simulink model "AFO_Hopf__sim1"  (R2020a)
settings: Solver=ode4  StartTime=0.0  StopTime=20  FixedStep=0.01  RelTol=1e-3
PreLoadFcn:
  | addpath(genpath('./DMP_AFO_simulink'), genpath('./my_util'))
libraries: simulink x1
settings Model: Creator=12927  LastModifiedBy=12927

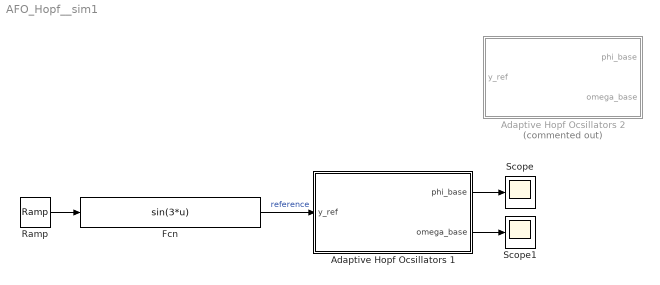
== system AFO_Hopf__sim1 ==
  Adaptive Hopf Ocsillators 1 : Subsystem
  Adaptive Hopf Ocsillators 2 : Subsystem  Commented=on
  Fcn : Fcn  Expr=sin(3*u)
  Ramp : simulink/Sources/Ramp  slope=1  start=0  InitialOutput=0
  Scope : Scope
  Scope1 : Scope
  wires:
  Ramp/1 -> Fcn/1
  Fcn/1 -> Adaptive Hopf Ocsillators 1/1(y_ref)  "reference"
  Adaptive Hopf Ocsillators 1/1(phi_base) -> Scope/1
  Adaptive Hopf Ocsillators 1/2(omega_base) -> Scope1/1

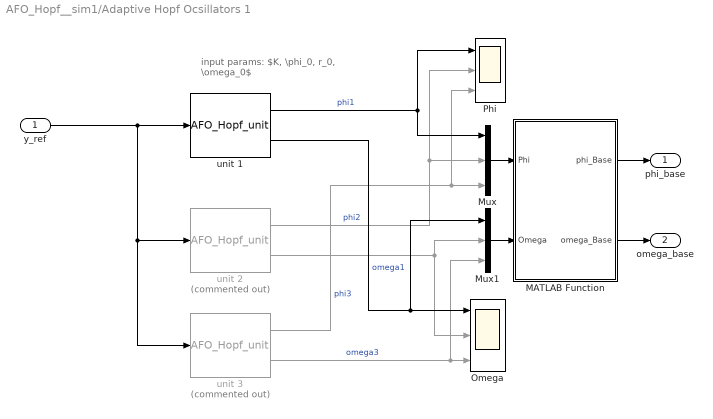
== system AFO_Hopf__sim1/Adaptive Hopf Ocsillators 1 ==
  note: input params:
      | $K, \phi_0, r_0, \omega_0$
  y_ref : Inport
  MATLAB Function : MATLAB Function  TreatAsAtomicUnit=on
  Mux : Mux  Inputs=3
  Mux1 : Mux  Inputs=3
  Omega : Scope  NumInputPorts=3
  Phi : Scope  NumInputPorts=3
  unit 1 : M-S-Function  FunctionName=AFO_Hopf_unit  Parameters=2,0,1,1
  unit 2 : M-S-Function  Commented=on  FunctionName=AFO_Hopf_unit  Parameters=10,0,1,1
  unit 3 : M-S-Function  Commented=on  FunctionName=AFO_Hopf_unit  Parameters=10,0,2,1
  phi_base : Outport
  omega_base : Outport  Port=2
  wires:
  unit 3/2 -> Omega/3, Mux1/3  "omega3"
  MATLAB Function/1(phi_Base) -> phi_base/1
  unit 2/1 -> Phi/2, Mux/2  "phi2"
  unit 2/2 -> Omega/2, Mux1/2
  Mux/1 -> MATLAB Function/1(Phi)
  unit 3/1 -> Mux/3, Phi/3  "phi3"
  Mux1/1 -> MATLAB Function/2(Omega)
  unit 1/1 -> Mux/1, Phi/1  "phi1"
  unit 1/2 -> Omega/1, Mux1/1  "omega1"
  MATLAB Function/2(omega_Base) -> omega_base/1
  y_ref/1 -> unit 1/1, unit 2/1, unit 3/1

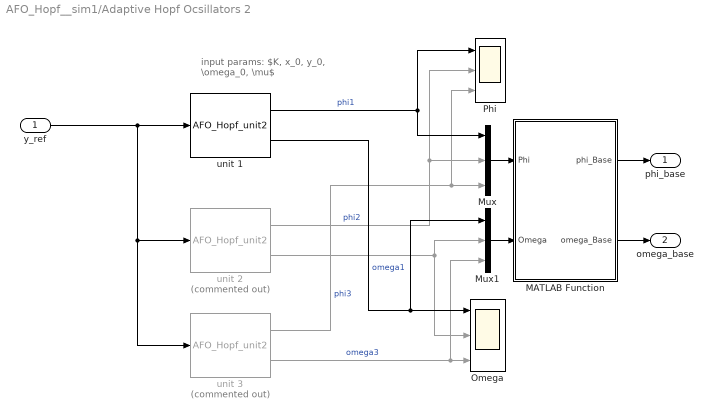
== system AFO_Hopf__sim1/Adaptive Hopf Ocsillators 2 ==
  note: input params:
      | $K, x_0, y_0, \omega_0, \mu$
  y_ref : Inport
  MATLAB Function : MATLAB Function  TreatAsAtomicUnit=on
  Mux : Mux  Inputs=3
  Mux1 : Mux  Inputs=3
  Omega : Scope  NumInputPorts=3
  Phi : Scope  NumInputPorts=3
  unit 1 : M-S-Function  FunctionName=AFO_Hopf_unit2  Parameters=5,1,0,1,1
  unit 2 : M-S-Function  Commented=on  FunctionName=AFO_Hopf_unit2  Parameters=5,1,0,1,1
  unit 3 : M-S-Function  Commented=on  FunctionName=AFO_Hopf_unit2  Parameters=5,1,0,1,1
  phi_base : Outport
  omega_base : Outport  Port=2
  wires:
  unit 3/2 -> Omega/3, Mux1/3  "omega3"
  MATLAB Function/1(phi_Base) -> phi_base/1
  unit 2/1 -> Phi/2, Mux/2  "phi2"
  unit 2/2 -> Omega/2, Mux1/2
  Mux/1 -> MATLAB Function/1(Phi)
  unit 3/1 -> Mux/3, Phi/3  "phi3"
  Mux1/1 -> MATLAB Function/2(Omega)
  unit 1/1 -> Mux/1, Phi/1  "phi1"
  unit 1/2 -> Omega/1, Mux1/1  "omega1"
  MATLAB Function/2(omega_Base) -> omega_base/1
  y_ref/1 -> unit 1/1, unit 2/1, unit 3/1

== matlab function AFO_Hopf__sim1/Adaptive Hopf Ocsillators 1/MATLAB Function ==
  data: Phi input; phi_Base output; Omega input; omega_Base output
function [phi_Base, omega_Base] = selectBaseSignal(Phi, Omega)

index1 = find(Omega);
Phi = Phi(index1);
[omega_Base, indexMin] = min(Omega(index1)); 
phi_Base = Phi(indexMin);

== matlab function AFO_Hopf__sim1/Adaptive Hopf Ocsillators 2/MATLAB Function ==
  data: Phi input; phi_Base output; Omega input; omega_Base output
function [phi_Base, omega_Base] = selectBaseSignal(Phi, Omega)

index1 = find(Omega);
Phi = Phi(index1);
[omega_Base, indexMin] = min(Omega(index1)); 
phi_Base = Phi(indexMin);
